simulink model "LQRAirrefuelingYingHu_la"  (R2013a)
settings: Solver=ode45  StartTime=0.0  StopTime=100  RelTol=1e-3
values from neighbouring files (symbols this model uses):
  A_la = A([2,4,6,9,10,12,15,16],[2,4,6,9,10,12,15,16])    [F16NolinearModelRemoveWindControlData_low.m]    (also in F16_2003hiModelAutopilot.m; F16_2003hiModelAutopilot1.m; F16_2003hiModelAutopilot1_steadySys.m = A([4,6,9,10,12,15,16],[4,6,9,10,12,15,16]); LQR_Calc2_F16YingHu_lonAndLa.m = A_full(8:12,8:12))
  B_la = B([2,4,6,9,10,12,15,16],3:4)    [F16NolinearModelRemoveWindControlData_low.m]    (also in F16_2003hiModelAutopilot.m; F16_2003hiModelAutopilot1.m; F16_2003hiModelAutopilot1_steadySys.m = B([4,6,9,10,12,15,16],3:4); LQR_Calc2_F16YingHu_lonAndLa.m = B_full(8:12,3:4))
  C_yd = [1   0   0   0   0]    [LQR_Calc2_F16YingHu_lonAndLa.m]
  Ki_la = -k_la(:,9)    [F16NolinearModelRemoveWindControlData_low.m]    (also in F16_2003hiModelAutopilot.m; F16_2003hiModelAutopilot1.m; LQR_Calc2_F16YingHu_lonAndLa.m = -k_la(:,6))
  Kp_la = k_la(:,1:8)    [F16NolinearModelRemoveWindControlData_low.m]    (also in F16_2003hiModelAutopilot.m; F16_2003hiModelAutopilot1.m; F16_2003hiModelAutopilot1_steadySys.m = k_la; LQR_Calc2_F16YingHu_lonAndLa.m = k_la(:,1:5))
settings Model: Creator=Dai  LastModifiedBy=Dai

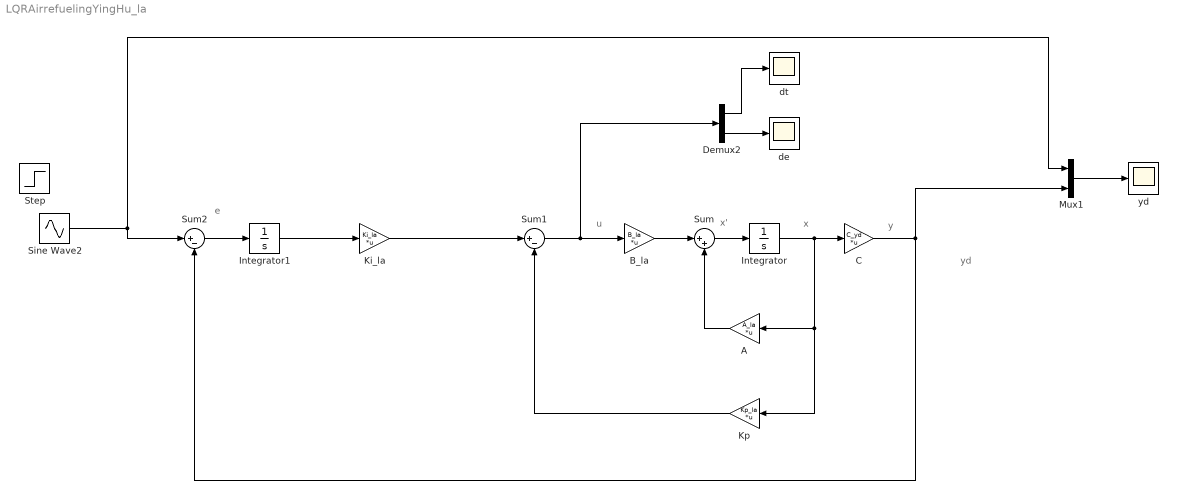
== system LQRAirrefuelingYingHu_la ==
  note: x
  note: x'
  note: y
  note: u
  note: yd
  note: e
  A : Gain  Gain=A_la  Multiplication=Matrix(K*u) (u vector)
  B_la : Gain  Gain=B_la  Multiplication=Matrix(K*u) (u vector)
  C : Gain  Gain=C_yd  Multiplication=Matrix(K*u) (u vector)
  Demux2 : Demux  Outputs=2
  Integrator : Integrator
  Integrator1 : Integrator
  Ki_la : Gain  Gain=Ki_la  Multiplication=Matrix(K*u) (u vector)
  Kp : Gain  Gain=Kp_la  Multiplication=Matrix(K*u) (u vector)
  Mux1 : Mux  Inputs=2
  Sine Wave2 : Sin  Amplitude=5  Frequency=0.05  SampleTime=0
  Step : Step  Time=5  After=5  SampleTime=0
  Sum : Sum  Inputs=|++
  Sum1 : Sum  Inputs=|+-
  Sum2 : Sum  Inputs=|+-
  de : Scope
      settings: SaveName=ScopeData3
  dt : Scope
      settings: SaveName=ScopeData2
  yd : Scope
  wires:
  Integrator/1 -> C/1, A/1, Kp/1
  B_la/1 -> Sum/1
  Sum/1 -> Integrator/1
  A/1 -> Sum/2
  Ki_la/1 -> Sum1/1
  C/1 -> Mux1/2, Sum2/2
  Sine Wave2/1 -> Mux1/1, Sum2/1
  Mux1/1 -> yd/1
  Kp/1 -> Sum1/2
  Sum2/1 -> Integrator1/1
  Demux2/1 -> dt/1
  Demux2/2 -> de/1
  Sum1/1 -> B_la/1, Demux2/1
  Integrator1/1 -> Ki_la/1
